simulink model "MBD_ques8"  (R2020a)
settings: Solver=VariableStepAuto  StartTime=0.0  StopTime=10.0  RelTol=1e-3
settings Model: Creator=DELL  LastModifiedBy=DELL

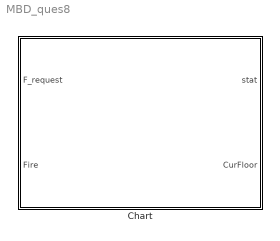
== system MBD_ques8 ==
  Chart : Stateflow chart  TreatAsAtomicUnit=on

== stateflow chart MBD_ques8/Chart ==
  state LiftOn
    state GroundFloor
      entry:
      stat=1;
      during:
      CurFloor=0;
      FloorOperation(CurFloor);
      exit:
      stat=0;
      after(20,sec);
    state FirstFloor
      entry:
      stat=1;
      during:
      CurFloor=1;
      FloorOperation(CurFloor);
      exit:
      stat=0;
      after(20,sec);
    state SecondFloor
      entry:
      stat=1;
      during:
      CurFloor=2;
      FloorOperation(CurFloor);
      exit:
      stat=0;
      after(20,sec);
    state ThirdFloor
      entry:
      stat=1;
      during:
      CurFloor=3;
      FloorOperation(CurFloor);
      exit:
      stat=0;
      after(20,sec);
    state FourthFloor
      entry:
      stat=1;
      during:
      CurFloor=4;
      FloorOperation(CurFloor);
      exit:
      stat=0;
      after(20,sec);
    state FifthFloor
      entry:
      stat=1;
      during:
      CurFloor=5;
      FloorOperation(CurFloor);
      exit:
      stat=0;
      after(20,sec);
    (default) -> GroundFloor
    GroundFloor -> FirstFloor : FloorUp
    FirstFloor -> GroundFloor [order 2] : FloorDown
    FirstFloor -> SecondFloor [order 1] : FloorUp
    SecondFloor -> FirstFloor [order 2] : FloorDown
    SecondFloor -> ThirdFloor [order 1] : FloorUp
    ThirdFloor -> SecondFloor [order 2] : FloorDown
    ThirdFloor -> FourthFloor [order 1] : FloorUp
    FourthFloor -> ThirdFloor [order 2] : FloorDown
    FourthFloor -> FifthFloor [order 1] : FloorUp
    FifthFloor -> FourthFloor : FloorDown
  state LiftOff
    en:
    stat=0;
  state AlarmSet
    (default) -> (junction 97) : {alarmStat=Fire;}
    (junction 97) -> (junction 100)
    (junction 100) -> (junction 102) [order 1] : [1]
    (junction 102) -> (junction 106) [order 2] : [alarmStat==1]{send(OpOff);}
    (junction 100) -> (junction 113) [order 2]
    (junction 102) -> (junction 104) [order 1] : [alarmStat==0]{send(OpOn);}
    (junction 106) -> (junction 108)
    (junction 108) -> (junction 104)
  state y = FloorOperation(floor) [function]
    (default) -> (junction 60)
    (junction 60) -> (junction 59) [order 3] : [F_request<floor]{
        | send(FloorDown);
        | disp('Down');}
    (junction 60) -> (junction 58) [order 1] : [F_request>floor]{
        | send(FloorUp);
        | disp('Up');}
    (junction 58) -> (junction 65)
    (junction 60) -> (junction 62) [order 2] : [F_request==floor]{
        | disp('CurrentFloor');}
    (junction 59) -> (junction 66)
    (junction 65) -> (junction 62)
    (junction 66) -> (junction 62)
    (junction 62) -> (junction 52)
  (default) -> LiftOn
  LiftOff -> LiftOn : [Fire==0]
  LiftOn -> LiftOff : [Fire==1]
  data: floor function_input; y function_output; stat output; CurFloor output; F_request input; Fire input; alarmStat local
  events: FloorUp local FUNCTION_CALL_EVENT; FloorDown local FUNCTION_CALL_EVENT; OpOn local FUNCTION_CALL_EVENT; OpOff local FUNCTION_CALL_EVENT
